simulink model "SFlowDiscrete"  (R2017a)
settings: Solver=VariableStepAuto  StartTime=0.0  StopTime=0.2  MaxStep=1e-6  RelTol=1e-3
values from neighbouring files (symbols this model uses):
  H1 = tf(n11,d11)    [funcionestransf.m]
  H1d = c2d(H1,Ts)    [funcionestransf.m]
  H2 = tf(n12,d12)    [funcionestransf.m]
  H2d = c2d(H2,Ts)    [funcionestransf.m]
  H3 = tf(n13,d13)    [funcionestransf.m]
  H3d = c2d(H3,Ts)    [funcionestransf.m]
  H4 = tf(n14,d14)    [funcionestransf.m]
  H4d = c2d(H4,Ts)    [funcionestransf.m]
  Ts = Ts_mpc    (= 0.03)    [Discretizer.m]    (also in funcionestransf.m = 0.00024)
libraries: simulink_extras x4
settings Model: Creator=erich  LastModifiedBy=Administrador

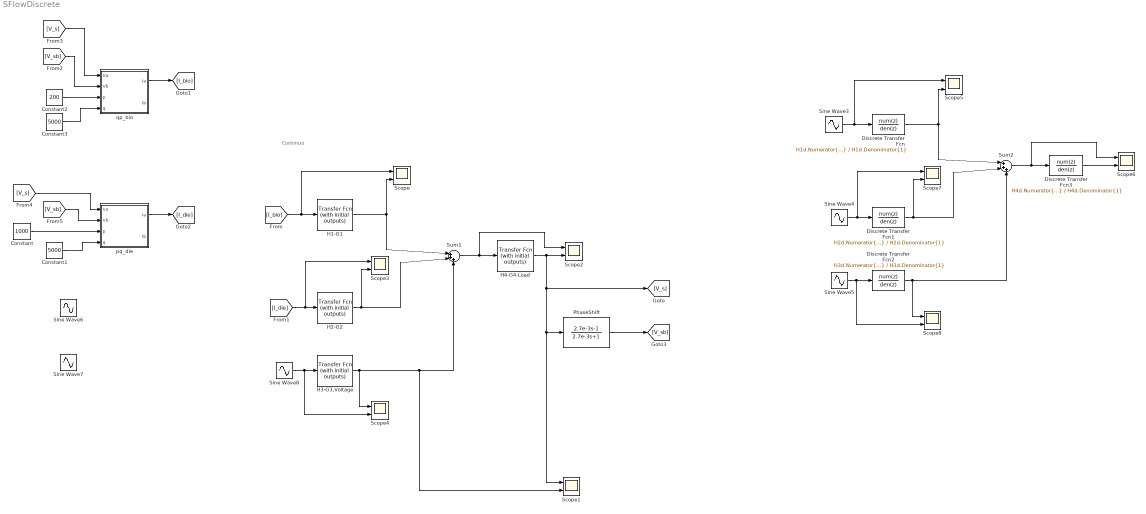
== system SFlowDiscrete ==
  note: Continuo
  Constant : Constant  Value=1000
  Constant1 : Constant  Value=5000
  Constant2 : Constant  Value=200
  Constant3 : Constant  Value=5000
  Discrete Transfer Fcn : DiscreteTransferFcn  Numerator=H1d.Numerator{1}  Denominator=H1d.Denominator{1}  SampleTime=Ts
  Discrete Transfer Fcn1 : DiscreteTransferFcn  Numerator=H2d.Numerator{1}  Denominator=H2d.Denominator{1}  SampleTime=Ts
  Discrete Transfer Fcn2 : DiscreteTransferFcn  Numerator=H3d.Numerator{1}  Denominator=H3d.Denominator{1}  SampleTime=Ts
  Discrete Transfer Fcn3 : DiscreteTransferFcn  Numerator=H4d.Numerator{1}  Denominator=H4d.Denominator{1}  SampleTime=Ts
  H1-G1 : simulink_extras/Additional Linear/Transfer Fcn (with initial outputs)  N=H1.Numerator{1}  D=H1.Denominator{1}  Y0=0  U0=0
  H2-G2 : simulink_extras/Additional Linear/Transfer Fcn (with initial outputs)  N=H2.Numerator{1}  D=H2.Denominator{1}  Y0=0  U0=0
  H3-G3,Voltage : simulink_extras/Additional Linear/Transfer Fcn (with initial outputs)  N=H3.Numerator{1}  D=H3.Denominator{1}  Y0=0  U0=0
  H4-G4-Load : simulink_extras/Additional Linear/Transfer Fcn (with initial outputs)  N=H4.Numerator{1}  D=H4.Denominator{1}  Y0=0  U0=0
  PhaseShift : TransferFcn  Numerator=[2.7e-3 -1]  Denominator=[2.7e-3 1]
  Scope{,1..8} (9 alike) : Scope  NumInputPorts=2
  Sine Wave{3..4,6..7} (4 alike) : Sin  Amplitude=10  Frequency=2*pi*60  SampleTime=0
  Sine Wave5 : Sin  Amplitude=170  Frequency=2*pi*60  SampleTime=0
  Sine Wave8 : Sin  Amplitude=170  Frequency=2*pi*60  SampleTime=0
  Sum1 : Sum  Inputs=|+++
  Sum2 : Sum  Inputs=|+++
  pq_die : MATLAB Function  TreatAsAtomicUnit=on
  qp_bio : MATLAB Function  TreatAsAtomicUnit=on
  wires:
  [I_bio] -> Scope/1, H1-G1/1
  H1-G1/1 -> Sum1/1, Scope/2
  H2-G2/1 -> Scope3/2, Sum1/2
  [I_die] -> Scope3/1, H2-G2/1
  Sine Wave8/1 -> Scope4/2, H3-G3,Voltage/1
  H3-G3,Voltage/1 -> Scope4/1, Scope1/2, Sum1/3
  Sum1/1 -> Scope2/1, H4-G4-Load/1
  H4-G4-Load/1 -> Scope1/1, PhaseShift/1, [V_s], Scope2/2
  Discrete Transfer Fcn3/1 -> Scope6/2
  Sum2/1 -> Discrete Transfer Fcn3/1, Scope6/1
  Discrete Transfer Fcn/1 -> Sum2/1, Scope5/2
  Sine Wave5/1 -> Discrete Transfer Fcn2/1, Scope8/2
  Discrete Transfer Fcn1/1 -> Scope7/2, Sum2/2
  Sine Wave4/1 -> Discrete Transfer Fcn1/1, Scope7/1
  Sine Wave3/1 -> Discrete Transfer Fcn/1, Scope5/1
  Discrete Transfer Fcn2/1 -> Scope8/1, Sum2/3
  qp_bio/1(Ia) -> [I_bio]
  pq_die/1(Ia) -> [I_die]
  PhaseShift/1 -> [V_sb]
  [V_sb] -> qp_bio/2(Vb)
  [V_s] -> qp_bio/1(Va)
  [V_s] -> pq_die/1(Va)
  [V_sb] -> pq_die/2(Vb)
  Constant/1 -> pq_die/3(p)
  Constant1/1 -> pq_die/4(q)
  Constant3/1 -> qp_bio/4(q)
  Constant2/1 -> qp_bio/3(p)

== matlab function SFlowDiscrete/pq_die ==
  data: Va input; Ia output; Vb input; p input; q input; Ib output
function [Ia, Ib] = fcn(Va, Vb, p, q)
%#codegen

% divide by zero protection
if(abs((Va^2+Vb^2))<=1000*eps(0))
    det = 1/eps(0);
else
    det = 1/(Va^2+Vb^2); % constante auxiliar
end;
%det = 1/(Va^2+Vb^2);

Mat = det*[Va Vb; Vb -Va];
Iab = Mat*[2*p;2*q];

Iaaux = Iab(1);
Ibaux = Iab(2);

ilim=1e3;

if(Iaaux>ilim)
    Iaaux=ilim;
end;
if(Iaaux<-ilim)
    Iaaux =-ilim;    
end;

if(isnan(Iaaux))
    Iaaux=0;
end;
%-----------------


if(Ibaux>ilim)
    Ibaux=ilim;
end;
if(Ibaux<-ilim)
    Ibaux =-ilim;    
end;

if(isnan(Ibaux))
    Ibaux=0;
end;
%-----------------


Ia = Iaaux;
Ib = Ibaux;

== matlab function SFlowDiscrete/qp_bio ==
  data: Va input; Ia output; Vb input; p input; q input; Ib output
function [Ia, Ib] = fcn(Va, Vb, p, q)
%#codegen

% divide by zero protection
if(abs((Va^2+Vb^2))<=1000*eps(0))
    det = 1/eps(0);
else
    det = 1/(Va^2+Vb^2); % constante auxiliar
end;
%det = 1/(Va^2+Vb^2);

Mat = det*[Va Vb; Vb -Va];
Iab = Mat*[2*p;2*q];

Iaaux = Iab(1);
Ibaux = Iab(2);

ilim=1e3;

if(Iaaux>ilim)
    Iaaux=ilim;
end;
if(Iaaux<-ilim)
    Iaaux =-ilim;    
end;

if(isnan(Iaaux))
    Iaaux=0;
end;
%-----------------


if(Ibaux>ilim)
    Ibaux=ilim;
end;
if(Ibaux<-ilim)
    Ibaux =-ilim;    
end;

if(isnan(Ibaux))
    Ibaux=0;
end;
%-----------------


Ia = Iaaux;
Ib = Ibaux;
